simulink model "second"  (R2016a)
settings: Solver=VariableStepAuto  StartTime=0.0  StopTime=10.0  RelTol=1e-3
settings Model: Creator=kypis  LastModifiedBy=kypis

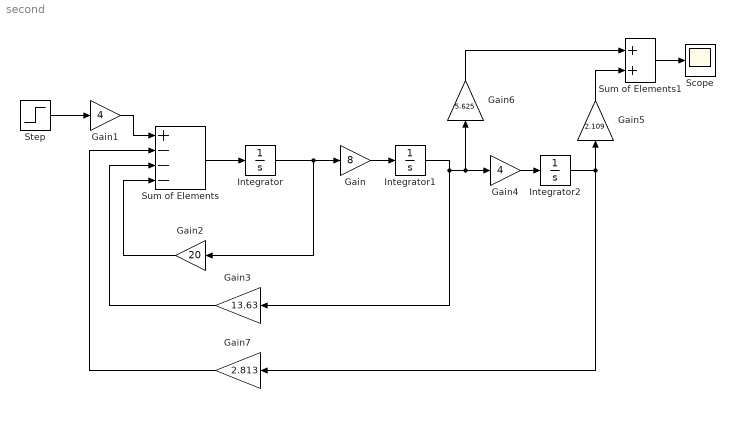
== system second ==
  Gain : Gain  Gain=8
  Gain1 : Gain  Gain=4
  Gain2 : Gain  Gain=20
  Gain3 : Gain  Gain=13.63
  Gain4 : Gain  Gain=4
  Gain5 : Gain  Gain=2.109
  Gain6 : Gain  Gain=5.625
  Gain7 : Gain  Gain=2.813
  Integrator : Integrator
  Integrator1 : Integrator
  Integrator2 : Integrator
  Scope : Scope
  Step : Step  Time=0  SampleTime=0
  Sum of Elements : Sum  Inputs=+---
  Sum of Elements1 : Sum
  wires:
  Step/1 -> Gain1/1
  Gain1/1 -> Sum of Elements/1
  Sum of Elements/1 -> Integrator/1
  Integrator/1 -> Gain2/1, Gain/1
  Gain2/1 -> Sum of Elements/4
  Gain/1 -> Integrator1/1
  Integrator1/1 -> Gain3/1, Gain4/1, Gain6/1
  Gain3/1 -> Sum of Elements/3
  Gain4/1 -> Integrator2/1
  Integrator2/1 -> Gain7/1, Gain5/1
  Gain5/1 -> Sum of Elements1/2
  Sum of Elements1/1 -> Scope/1
  Gain6/1 -> Sum of Elements1/1
  Gain7/1 -> Sum of Elements/2
